simulink model "state_machine"  (R2017b)
settings: Solver=FixedStepDiscrete  StartTime=0.0  StopTime=inf  FixedStep=0.00005  RelTol=1e-3
libraries: dspnetwork x5, simulink_extras x1, etargetslib x1, xpcrtudplib x1
settings Model: Creator=exo-hand  LastModifiedBy=Ronda
settings RTWCC: TemplateMakefile=RTW.MSVCBuild  Description=Create Visual C/C++ Solution File for Simulink Coder

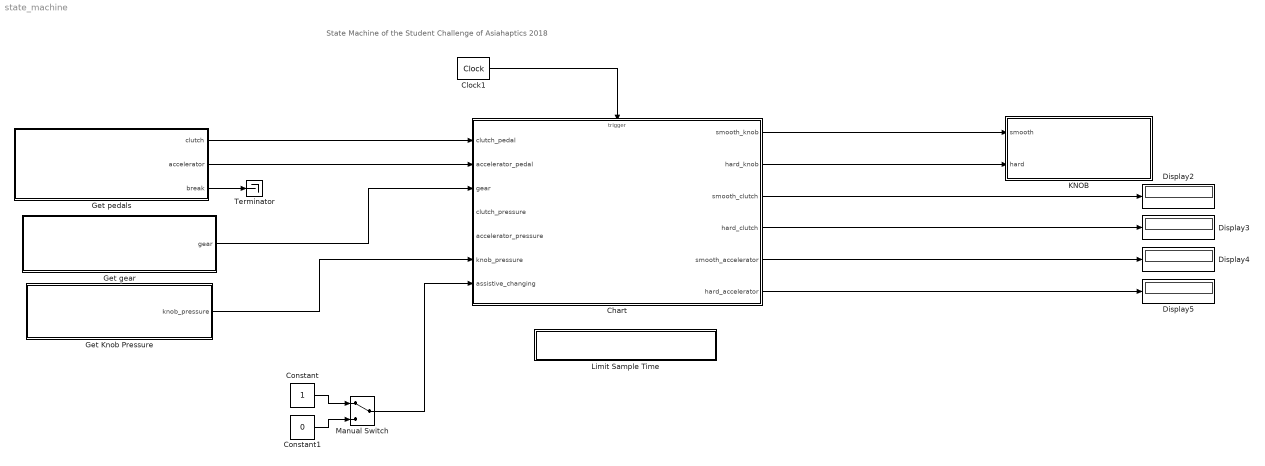
== system state_machine ==
  note: State Machine of the Student Challenge of Asiahaptics 2018
  Chart : Stateflow chart  TreatAsAtomicUnit=on
  Clock1 : simulink_extras/Flip Flops/Clock  period=0.005
  Constant : Constant  OutDataTypeStr=int16
  Constant1 : Constant  Value=0  OutDataTypeStr=int16
  Display{2..5} (4 alike) : Display
  Get Knob Pressure : Subsystem
  Get gear : Subsystem
  Get pedals : Subsystem
  KNOB : Subsystem
  Limit Sample Time : Subsystem
  Manual Switch : ManualSwitch
  Terminator : Terminator
  wires:
  Clock1/1 -> Chart/Trigger
  Chart/3(smooth_clutch) -> Display2/1
  Chart/4(hard_clutch) -> Display3/1
  Chart/5(smooth_accelerator) -> Display4/1
  Chart/6(hard_accelerator) -> Display5/1
  Constant/1 -> Manual Switch/1
  Constant1/1 -> Manual Switch/2
  Manual Switch/1 -> Chart/7(assistive_changing)
  Get pedals/1(clutch) -> Chart/1(clutch_pedal)
  Get pedals/2(accelerator) -> Chart/2(accelerator_pedal)
  Get pedals/3("break ") -> Terminator/1
  Get gear/1(gear) -> Chart/3(gear)
  Chart/1(smooth_knob) -> KNOB/1(smooth)
  Chart/2(hard_knob) -> KNOB/2(hard)
  Get Knob Pressure/1(knob_pressure) -> Chart/6(knob_pressure)

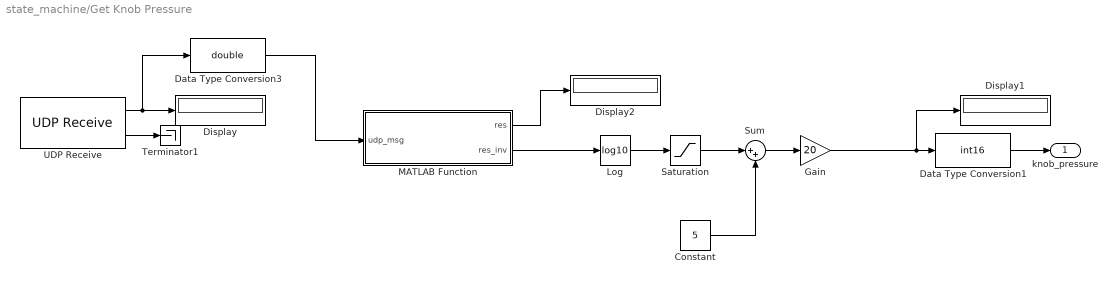
== system state_machine/Get Knob Pressure ==
  Constant : Constant  Value=5
  Data Type Conversion1 : DataTypeConversion  OutDataTypeStr=int16
  Data Type Conversion3 : DataTypeConversion  OutDataTypeStr=double
  Display : Display
  Display1 : Display
  Display2 : Display
  Gain : Gain  Gain=20
  Log : Math  Operator=log10  SaturateOnIntegerOverflow=on
  MATLAB Function : MATLAB Function  TreatAsAtomicUnit=on
  Saturation : Saturate  UpperLimit=0  LowerLimit=-5
  Sum : Sum  Inputs=|++
  Terminator1 : Terminator
  UDP Receive : dspnetwork/UDP Receive  localURL='0.0.0.0'  localPort=30100  remoteURL='192.168.0.30'  remotePort=-1  recvBufferSize=2  dims=1  signalDatatype=int16  isVarSize=off  showBlockingTime=off  blockingTime=0  sampletime=0.01  blockPlatform=[]
      settings: SourceProductName=DSP System Toolbox  SourceProductBaseCode=DS
  knob_pressure : Outport
  wires:
  UDP Receive/2 -> Terminator1/1
  UDP Receive/1 -> Data Type Conversion3/1, Display/1
  Log/1 -> Saturation/1
  Data Type Conversion1/1 -> knob_pressure/1
  MATLAB Function/2(res_inv) -> Log/1
  Gain/1 -> Display1/1, Data Type Conversion1/1
  MATLAB Function/1(res) -> Display2/1
  Data Type Conversion3/1 -> MATLAB Function/1(udp_msg)
  Saturation/1 -> Sum/1
  Sum/1 -> Gain/1
  Constant/1 -> Sum/2

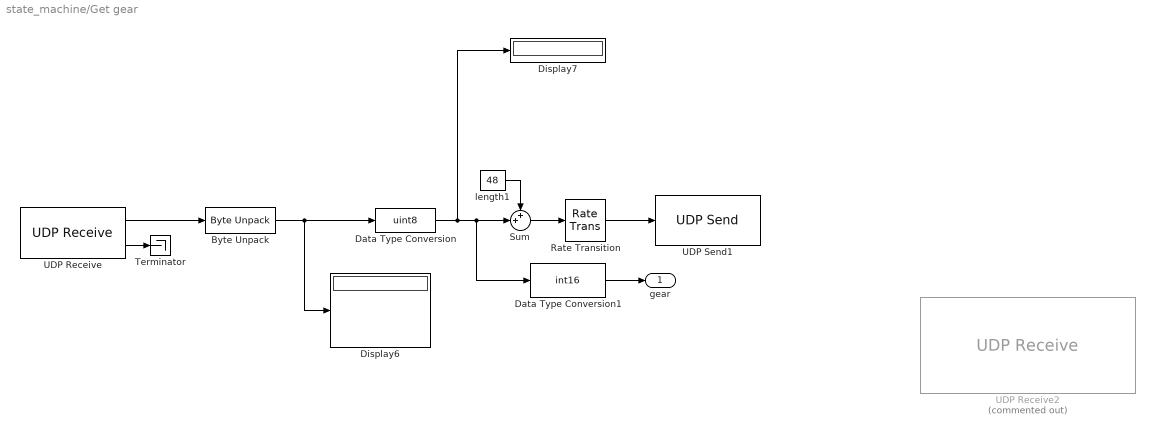
== system state_machine/Get gear ==
  Byte Unpack : etargetslib/Byte Unpack  dimensions={[1]}  datatypes={'single'}  byteAlign=1
  Data Type Conversion : DataTypeConversion  OutDataTypeStr=uint8
  Data Type Conversion1 : DataTypeConversion  OutDataTypeStr=int16
  Display6 : Display
  Display7 : Display
  Rate Transition : RateTransition  OutPortSampleTime=0.02
  Sum : Sum  Inputs=++|
  Terminator : Terminator
  UDP Receive : dspnetwork/UDP Receive  localURL='0.0.0.0'  localPort=20002  remoteURL='192.168.0.2'  remotePort=-1  recvBufferSize=4  dims=4  signalDatatype=uint8  isVarSize=off  showBlockingTime=off  blockingTime=0  sampletime=0.00005  blockPlatform=[]
      settings: SourceProductName=DSP System Toolbox  SourceProductBaseCode=DS
  UDP Receive2 : xpcrtudplib/UDP Receive  Commented=on  ipAddressVal=Use host-target connection  localPort=20002  rcvWidth=4  rcvFmAny=off  fmAddress=192.168.0.2  maxUDPQueue=8  sampleTime=0.00005
      settings: SourceProductName=Simulink Real-Time
  UDP Send1 : dspnetwork/UDP Send  remoteURL='127.0.0.1'  remotePort=25001  localURL='0.0.0.0'  localPortSource=Automatically determine  localPort=-1  sampletime=-1  blockPlatform=[]  separateLengthPort=0
      settings: SourceProductName=DSP System Toolbox  SourceProductBaseCode=DS
  length1 : Constant  Value=48  OutDataTypeStr=uint8
  gear : Outport
  wires:
  UDP Receive/2 -> Terminator/1
  Sum/1 -> Rate Transition/1
  Byte Unpack/1 -> Display6/1, Data Type Conversion/1
  Rate Transition/1 -> UDP Send1/1
  UDP Receive/1 -> Byte Unpack/1
  length1/1 -> Sum/1
  Data Type Conversion/1 -> Data Type Conversion1/1, Sum/2, Display7/1
  Data Type Conversion1/1 -> gear/1

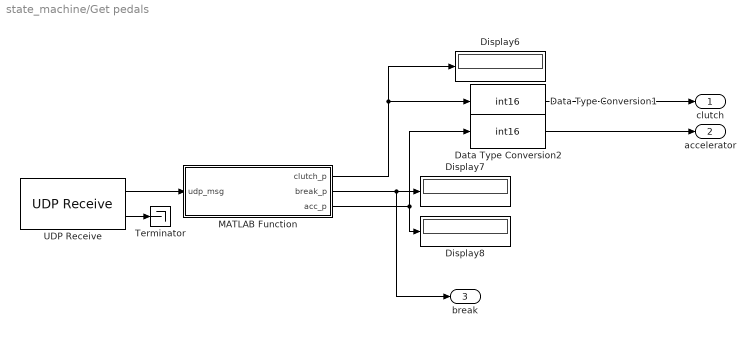
== system state_machine/Get pedals ==
  Data Type Conversion1 : DataTypeConversion  OutDataTypeStr=int16
  Data Type Conversion2 : DataTypeConversion  OutDataTypeStr=int16
  Display6 : Display
  Display7 : Display
  Display8 : Display
  MATLAB Function : MATLAB Function  TreatAsAtomicUnit=on
  Terminator : Terminator
  UDP Receive : dspnetwork/UDP Receive  localURL='0.0.0.0'  localPort=28000  remoteURL='127.0.0.1'  remotePort=-1  recvBufferSize=20  dims=15  signalDatatype=uint8  isVarSize=off  showBlockingTime=off  blockingTime=0  sampletime=0.02  blockPlatform=[]
      settings: SourceProductName=DSP System Toolbox  SourceProductBaseCode=DS
  clutch : Outport
  accelerator : Outport  Port=2
  "break " : Outport  Port=3
  wires:
  Data Type Conversion1/1 -> clutch/1
  MATLAB Function/1(clutch_p) -> Data Type Conversion1/1, Display6/1
  MATLAB Function/2(break_p) -> "break "/1, Display7/1
  UDP Receive/1 -> MATLAB Function/1(udp_msg)
  MATLAB Function/3(acc_p) -> Data Type Conversion2/1, Display8/1
  UDP Receive/2 -> Terminator/1
  Data Type Conversion2/1 -> accelerator/1

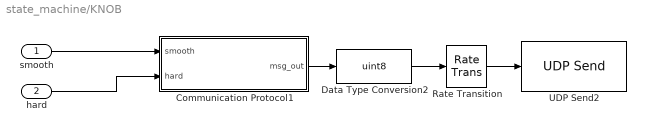
== system state_machine/KNOB ==
  smooth : Inport
  hard : Inport  Port=2
  Communication Protocol1 : MATLAB Function  TreatAsAtomicUnit=on
  Data Type Conversion2 : DataTypeConversion  OutDataTypeStr=uint8
  Rate Transition : RateTransition  OutPortSampleTime=0.01
  UDP Send2 : dspnetwork/UDP Send  remoteURL='192.168.0.30'  remotePort=29500  localURL='0.0.0.0'  localPortSource=Automatically determine  localPort=-1  sampletime=-1  blockPlatform=[]  separateLengthPort=0
      settings: SourceProductName=DSP System Toolbox  SourceProductBaseCode=DS
  wires:
  Communication Protocol1/1(msg_out) -> Data Type Conversion2/1
  Rate Transition/1 -> UDP Send2/1
  Data Type Conversion2/1 -> Rate Transition/1
  smooth/1 -> Communication Protocol1/1(smooth)
  hard/1 -> Communication Protocol1/2(hard)

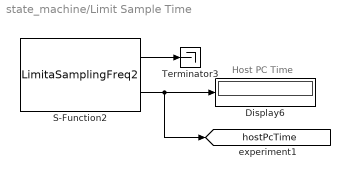
== system state_machine/Limit Sample Time ==
  note: Host PC Time
  Display6 : Display
  S-Function2 : S-Function  FunctionName=LimitaSamplingFreq2  Parameters=str2num(get_param(bdroot,'FixedStep'))  SFunctionDeploymentMode=off  EnableBusSupport=off
  Terminator3 : Terminator
  tag scope: hostPcTime=global
  wires:
  S-Function2/1 -> Terminator3/1
  S-Function2/2 -> [hostPcTime], Display6/1

== matlab function state_machine/Get Knob Pressure/MATLAB Function ==
  data: res output; udp_msg input; res_inv output
function [res,res_inv]  = get_FSR_resistance(udp_msg)
%% The function returns the value of the FSR resistance
% starting from the ADC value (the signal passes through a voltage divider
r_in = 1000, % Ohm
V_in = 4096; % ADC ticks
V_out = udp_msg; % ADC ticks

res = r_in * (V_in - V_out) / V_out;
res_inv = 1/res;
end

== matlab function state_machine/Get pedals/MATLAB Function ==
  data: udp_msg input; clutch_p output; break_p output; acc_p output
function [clutch_p, break_p, acc_p] = get_pedals(udp_msg)
%% The function provides the values of pression of the pedals
%  as an integer number between 0 and 100 (0 released, 100 completely
%  pressed)

clutch_p = 100 - (get_number(udp_msg(2))*100 + get_number(udp_msg(4))*10 + get_number(udp_msg(5)));
break_p = 100 - (get_number(udp_msg(7))*100 + get_number(udp_msg(9))*10 + get_number(udp_msg(10)));
acc_p = 100 - (get_number(udp_msg(12))*100 + get_number(udp_msg(14))*10 + get_number(udp_msg(15)));

end

function [number] = get_number(char)
    number = char - 48;
end

== stateflow chart state_machine/Chart ==
  settings: executeAtInitialization=1
  state CLUTCH_and_KNOB [parallel]
    settings: executionOrder=1
    state Gear_changing_process
      % This Part is assistive driving and can be deactivated if necessary
      state START
        % The system waits for the knob_action
        entry:smooth_knob
        exit:smooth_knob
      state Wait_for_gear_change
        state KNOB_1
          % The action of change starts
          % Neutral Gear
        state KNOB_3
          % The driver waits a lot to change
          entry:smooth_knob
          exit:smooth_knob
        KNOB_1 -> KNOB_3 : after(TIME_THRESHOLD,tick_in)
      state KNOB_2
        % The driver changes the gear
        entry:smooth_clutch
        exit:smooth_clutch
      (default) -> START
      START -> KNOB_1 : [gear==8]
      Wait_for_gear_change -> KNOB_2 : [gear<8]/{completed=true}
    state Wait_and_assist
      state WAIT
        entry: completed=true
      state Wait_knob
        state WAIT_FOR_KNOB
          % The driver should hold
          % the knob
        state CLUTCH_UNNECESSARY
          entry:hard_clutch
          exit:hard_clutch
        (default) -> WAIT_FOR_KNOB
        WAIT_FOR_KNOB -> CLUTCH_UNNECESSARY : [knob_pressure < KNOB_PRESSURE_TH & after(TIME_THRESHOLD,tick_in)]
      state KNOB_UNNECESSARY
        entry: hard_knob
        exit: hard_knob
      (default) -> WAIT
      WAIT -> Wait_knob [order 1] : [clutch_pedal > CLUTCH_THRESHOLD]/{completed=false}
      KNOB_UNNECESSARY -> WAIT [order 2] : [knob_pressure < KNOB_PRESSURE_TH]
      WAIT -> KNOB_UNNECESSARY [order 2] : [knob_pressure > KNOB_PRESSURE_TH & after(TIME_THRESHOLD,tick_in)]
      Wait_knob -> WAIT [order 2] : [clutch_pedal < CLUTCH_THRESHOLD]
    (default) -> Wait_and_assist
    Gear_changing_process -> WAIT : [clutch_pedal < CLUTCH_THRESHOLD]
    Wait_knob -> (junction 83) [order 1] : [knob_pressure > KNOB_PRESSURE_TH]
    (junction 83) -> Gear_changing_process [order 1] : [assistive_changing > 0]
    KNOB_UNNECESSARY -> (junction 83) [order 1] : [clutch_pedal > CLUTCH_THRESHOLD]/{completed=false}
    (junction 83) -> Wait_and_assist [order 2] : [assistive_changing < 1]
  state ACCELERATOR [parallel]
    settings: executionOrder=2
    state No_clutch
    state Error_accelerato
      entry: hard_accelerator
      exit: hard_accelerator
    No_clutch -> Error_accelerato : [completed==false & accelerator_pressure > ACCELERATOR_PRESSURE_TS]
    (default) -> No_clutch
    Error_accelerato -> No_clutch : [completed==true | accelerator_pressure < ACCELERATOR_PRESSURE_TS]
  data: clutch_pedal input int16; accelerator_pedal input int16; gear input int16; clutch_pressure input int16; accelerator_pressure input int16; knob_pressure input int16; CLUTCH_THRESHOLD constant int16 =50; TIME_THRESHOLD constant double =10; KNOB_PRESSURE_TH constant double =50; assistive_changing input int16; completed local boolean =true; ACCELERATOR_PRESSURE_TS constant int16 =10
  events: smooth_knob output EITHER_EDGE_EVENT; hard_knob output EITHER_EDGE_EVENT; smooth_clutch output EITHER_EDGE_EVENT; hard_clutch output EITHER_EDGE_EVENT; smooth_accelerator output EITHER_EDGE_EVENT; hard_accelerator output EITHER_EDGE_EVENT; tick_in input EITHER_EDGE_EVENT

== matlab function state_machine/KNOB/Communication Protocol1 ==
  data: smooth input; msg_out output; hard input
function msg_out  = generate_msg(smooth, hard)
%% The function generate the message depending on the state
msg = zeros(2,1);
if (smooth == 1)
    msg(1) = 1;
    msg(2) = 0;
else if (hard == 1)
        msg(1) = 2;
        msg(2) = 0;
    else
        msg(1) = 0;
        msg(2) = 0;
    end
end

msg_out = msg;
